simulink model "AllPass"  (R2020a)
settings: Solver=VariableStepAuto  StartTime=0.0  StopTime=100000.0  RelTol=1e-3
libraries: audiosources x1, dspsnks4 x1, dspsrcs4 x1
settings Model: Creator=ace  LastModifiedBy=ace

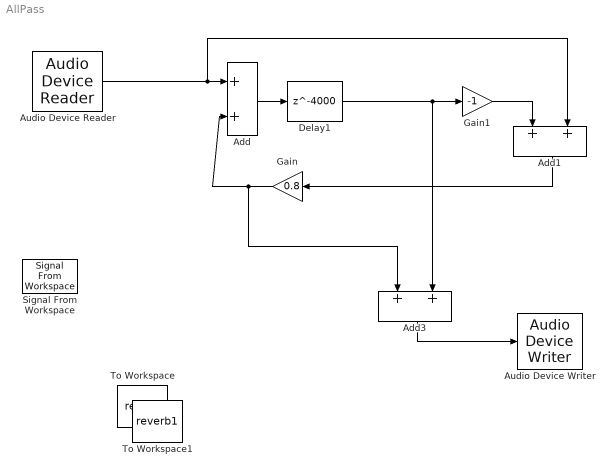
== system AllPass ==
  Add : Sum
  Add1 : Sum
  Add3 : Sum
  Audio Device Reader : audiosources/Audio Device Reader  Driver=CoreAudio  Device=Default  SampleRate=44100  NumChannels=1  SamplesPerFrame=1024  BitDepth=16-bit integer  NumBuffers=10  DefaultInputChannelMapping=on  InputChannelMapping=1:2  OutputNumOverrunSamples=off  OutputDataType=double  DriverIdx=5  DeviceWarnFlag=''
      settings: SourceProductBaseCode=AU
  Audio Device Writer : dspsnks4/Audio Device Writer  Driver=CoreAudio  Device=Default  InheritSampleRate=on  SampleRate=44100  BitDepth=16-bit integer  BufferSize=4096  NumBuffers=10  DefaultOutputChannelMapping=on  OutputChannelMapping=1:2  OutputNumUnderrunSamples=off  DriverIdx=5  DeviceWarnFlag=''
  Delay1 : Delay  DelayLength=4000  InputProcessing=Columns as channels (frame based)
  Gain : Gain  Gain=0.8
  Gain1 : Gain  Gain=-1
  Signal From Workspace : dspsrcs4/Signal From Workspace  X=Hello  Ts=1  nsamps=1  OutputAfterFinalValue=Setting to zero  ignoreOrWarnInputAndFrameLengths=off  OutputFrames=off
  To Workspace : ToWorkspace  VariableName=reverb  SampleTime=-1
      settings: Save2DSignal=2-D array (concatenate along first dimension)
  To Workspace1 : ToWorkspace  VariableName=reverb1  SampleTime=-1
      settings: Save2DSignal=2-D array (concatenate along first dimension)
  wires:
  Gain/1 -> Add/2, Add3/1
  Audio Device Reader/1 -> Add1/2, Add/1
  Add/1 -> Delay1/1
  Delay1/1 -> Gain1/1, Add3/2
  Gain1/1 -> Add1/1
  Add1/1 -> Gain/1
  Add3/1 -> Audio Device Writer/1
